simulink model "diagrama2_0"  (R2025a)
settings: Solver=ode4  StartTime=0.0  StopTime=20  FixedStep=1e-4  MaxStep=1e-3  RelTol=1e-3
InitFcn:
  | Np = 1;
  | Ns = 1;
  | Iscref = 1;
  | Voc = 1;
libraries: SignalEditorBlockLib x2, simulink x1
settings Model: Creator=BSLAY  LastModifiedBy=Rodri
settings SolverCC: InitialStep=1e-6
settings DebuggingCC: AlgebraicLoopMsg=none

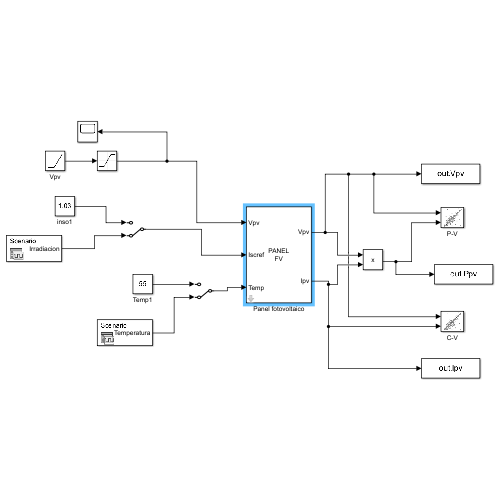
[thumbnail: Simulink's stored preview of the top-level diagram]
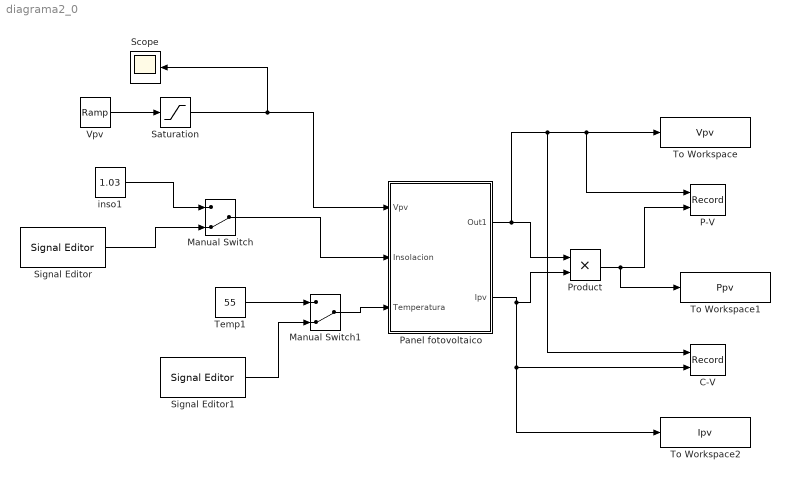
== system diagrama2_0 ==
  C-V : Record  NumPorts=2.0  FileSettingsInternal="{\"entries\":[{\"content\":{\"excelSettings\":{\"content\":{},\"type\":\"Streamout.ExcelSettings\"},\"parquetSettings\":{\"content\":{},\"type\":\"Streamout.ParquetSettings\"}},\"type\":\"Streamout.FileSettingStorage\",\"uuid\":\"\"}],\"packageUris\":[\"http:\\/\\/schema.mathworks.com\\/mf0\\/streamout_blocks\\/R2020a\"],\"version\":\"1.0\"}"  FrameSettings=[0, 0]  Layout=[1 1]  SignalsInternal="{\"entries\":[{\"content\":{\"signals\":[{\"content\":{\"blockPath\":[],\"dimensions\":[1],\"domain\":\"\",\"lineColor\":\"#7e2f8e\",\"lineWidth\":2,\"port\":1,\"sid\":[\"\"],\"signalID\":1,\"signalName\":\"Panel fotovoltaico:1\"},\"type\":\"RecordBlkView.Signal\",\"uuid\":\"\"},{\"content\":{\"blockPath\":[],\"dimensions\":[1],\"domain\":\"\",\"lineColor\":\"#77ac30\",\"lineWidth\":2,\"port\":2,\"sid\":[\"\"],\"signalID\":2,\"signalName\":\"Panel fotovoltaico:2\"},\"type\":\"RecordBlkView.Signal\",\"uuid\":\"\"}]},\"type\":\"RecordBlkView.InputSignals\",\"uuid\":\"\"}],\"packageUris\":[\"http:\\/\\/schema.mathworks.com\\/mf0\\/streamout_blocks\\/R2020a\"],\"version\":\"1.0\"}"  CompatibilityTag=XY
  Manual Switch : ManualSwitch  CurrentSetting=0
  Manual Switch1 : ManualSwitch  CurrentSetting=0
  P-V : Record  NumPorts=2.0  FileSettingsInternal="{\"entries\":[{\"content\":{\"excelSettings\":{\"content\":{},\"type\":\"Streamout.ExcelSettings\"},\"parquetSettings\":{\"content\":{},\"type\":\"Streamout.ParquetSettings\"}},\"type\":\"Streamout.FileSettingStorage\",\"uuid\":\"\"}],\"packageUris\":[\"http:\\/\\/schema.mathworks.com\\/mf0\\/streamout_blocks\\/R2020a\"],\"version\":\"1.0\"}"  FrameSettings=[0, 0]  Layout=[1 1]  SignalsInternal="{\"entries\":[{\"content\":{\"signals\":[{\"content\":{\"blockPath\":[],\"dimensions\":[1],\"domain\":\"\",\"lineColor\":\"#4dbeee\",\"lineWidth\":2,\"port\":1,\"sid\":[\"\"],\"signalID\":1,\"signalName\":\"Panel fotovoltaico:1\"},\"type\":\"RecordBlkView.Signal\",\"uuid\":\"\"},{\"content\":{\"blockPath\":[],\"dimensions\":[1],\"domain\":\"\",\"lineColor\":\"#a2142f\",\"lineWidth\":2,\"port\":2,\"sid\":[\"\"],\"signalID\":2,\"signalName\":\"Product\"},\"type\":\"RecordBlkView.Signal\",\"uuid\":\"\"}]},\"type\":\"RecordBlkView.InputSignals\",\"uuid\":\"\"}],\"packageUris\":[\"http:\\/\\/schema.mathworks.com\\/mf0\\/streamout_blocks\\/R2020a\"],\"version\":\"1.0\"}"  CompatibilityTag=XY
  Panel fotovoltaico : Subsystem  mask{Ns=36, Np=1, Corriente_en_corto_circuito=8.21, Voltaje_en_corto_circuito_abierto=37.3}
      mask prompts: Ns "Número de celdas en serie"; Np "Número de celdas en paralelo"; Corriente_en_corto_circuito "Iscref"; Voltaje_en_corto_circuito_abierto "Voc"
      mask Display:
      | disp('PANEL\nFV');
      | port_label('input', 1, 'Vpv');
      | port_label('input', 2, 'Iscref');
      | port_label('input', 3, 'Temp');
      | 
      | port_label('output', 1, 'Vpv');
      | port_label('output', 2, 'Ipv');
  Product : Product
  Saturation : Saturate  UpperLimit=40  LowerLimit=0
  Scope : Scope
      settings: ActiveDisplayYMinimum=-1  ActiveDisplayYMaximum=1
  Signal Editor : SignalEditorBlockLib/Signal Editor  FileName=Insolacion1.mat  ActiveScenario=Scenario  ActiveSignal=Irradiacion  IsBus=off  OutputBusObjectStr=Bus: BusObject  SampleTime=0  ZeroCross=off  OutputAfterFinalValue=Holding final value  Unit=W/m^2  PreserveSignalName=on  ApplySigPropsToAllScenarios=on  ApplySigPropsToAllSignals=off  SignalPropertySource=Dialog parameters
  Signal Editor1 : SignalEditorBlockLib/Signal Editor  FileName=Temperatura1.mat  ActiveScenario=Scenario  ActiveSignal=Temperatura  IsBus=off  OutputBusObjectStr=Bus: BusObject  SampleTime=0  ZeroCross=off  OutputAfterFinalValue=Holding final value  Unit=degC  PreserveSignalName=on  ApplySigPropsToAllScenarios=on  ApplySigPropsToAllSignals=off  SignalPropertySource=Dialog parameters
  Temp1 : Constant  Value=55
  To Workspace : ToWorkspace  VariableName=Vpv  SaveFormat=Timeseries  SampleTime=-1
  To Workspace1 : ToWorkspace  VariableName=Ppv  SaveFormat=Timeseries  SampleTime=-1
  To Workspace2 : ToWorkspace  VariableName=Ipv  SaveFormat=Timeseries  SampleTime=-1
  Vpv : simulink/Sources/Ramp  slope=-10/20  start=0  InitialOutput=10
  inso1 : Constant  Value=1.03
  wires:
  Manual Switch/1 -> Panel fotovoltaico/2(Insolacion)
  inso1/1 -> Manual Switch/1
  Manual Switch1/1 -> Panel fotovoltaico/3(Temperatura)
  Temp1/1 -> Manual Switch1/1
  Panel fotovoltaico/2(Ipv) -> To Workspace2/1, C-V/2, Product/2
  Panel fotovoltaico/1(Out1) -> C-V/1, P-V/1, To Workspace/1, Product/1
  Product/1 -> To Workspace1/1, P-V/2
  Signal Editor/1 -> Manual Switch/2
  Signal Editor1/1 -> Manual Switch1/2
  Vpv/1 -> Saturation/1
  Saturation/1 -> Scope/1, Panel fotovoltaico/1(Vpv)

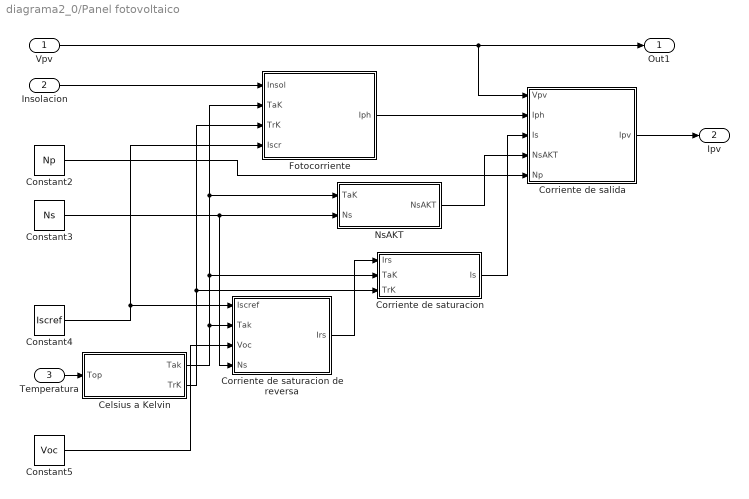
== system diagrama2_0/Panel fotovoltaico ==
  Vpv : Inport
  Insolacion : Inport  Port=2
  Temperatura : Inport  Port=3
  Celsius a Kelvin : Subsystem
  Constant2 : Constant  Value=Np
  Constant3 : Constant  Value=Ns
  Constant4 : Constant  Value=Iscref
  Constant5 : Constant  Value=Voc
  Corriente de salida : Subsystem
  Corriente de saturacion : Subsystem
  Corriente de saturacion de reversa : Subsystem
  Fotocorriente : Subsystem
  NsAKT : Subsystem
  Out1 : Outport
  Ipv : Outport  Port=2
  wires:
  Constant5/1 -> Corriente de saturacion de reversa/3(Voc)
  Corriente de salida/1(Ipv) -> Ipv/1
  Temperatura/1 -> Celsius a Kelvin/1(Top)
  Vpv/1 -> Corriente de salida/1(Vpv), Out1/1
  Fotocorriente/1(Iph) -> Corriente de salida/2(Iph)
  Insolacion/1 -> Fotocorriente/1(Insol)
  Constant3/1 -> Corriente de saturacion de reversa/4(Ns), NsAKT/2(Ns)
  Corriente de saturacion de reversa/1(Irs) -> Corriente de saturacion/1(Irs)
  Constant4/1 -> Corriente de saturacion de reversa/1(Iscref), Fotocorriente/4(Iscr)
  Constant2/1 -> Corriente de salida/5(Np)
  NsAKT/1(NsAKT) -> Corriente de salida/4(NsAKT)
  Corriente de saturacion/1(Is) -> Corriente de salida/3(Is)
  Celsius a Kelvin/1(Tak) -> Corriente de saturacion de reversa/2(Tak), Corriente de saturacion/2(TaK), NsAKT/1(TaK), Fotocorriente/2(TaK)
  Celsius a Kelvin/2(TrK) -> Corriente de saturacion/3(TrK), Fotocorriente/3(TrK)

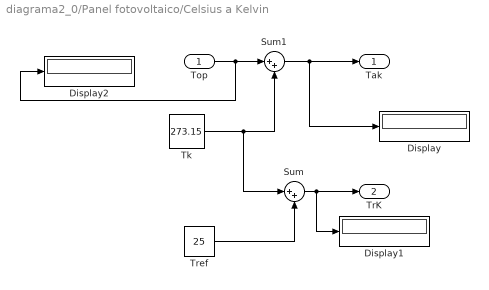
== system diagrama2_0/Panel fotovoltaico/Celsius a Kelvin ==
  Top : Inport
  Display : Display
  Display1 : Display
  Display2 : Display
  Sum : Sum  Inputs=|++
  Sum1 : Sum  Inputs=|++
  Tk : Constant  Value=273.15
  Tref : Constant  Value=25
  Tak : Outport
  TrK : Outport  Port=2
  wires:
  Sum/1 -> Display1/1, TrK/1
  Top/1 -> Display2/1, Sum1/1
  Tk/1 -> Sum/1, Sum1/2
  Sum1/1 -> Display/1, Tak/1
  Tref/1 -> Sum/2

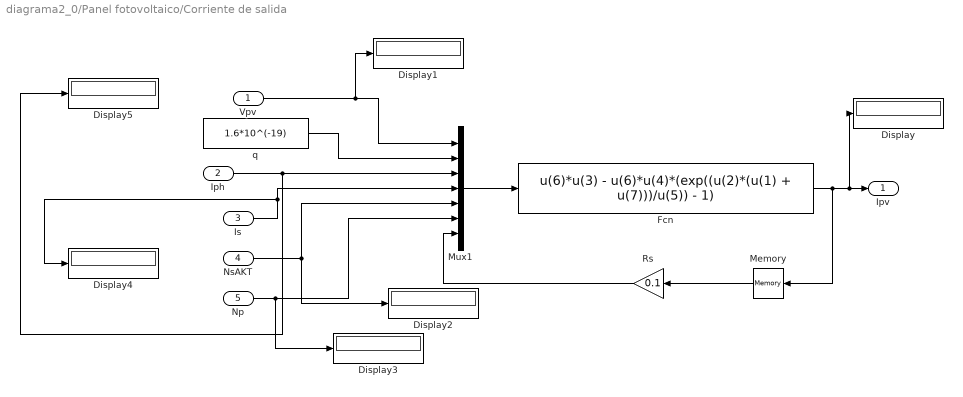
== system diagrama2_0/Panel fotovoltaico/Corriente de salida ==
  Vpv : Inport
  Iph : Inport  Port=2
  Is : Inport  Port=3
  NsAKT : Inport  Port=4
  Np : Inport  Port=5
  Display{,1..5} (6 alike) : Display
  "Fcn " : Fcn  Expr=u(6)*u(3) - u(6)*u(4)*(exp((u(2)*(u(1) + u(7)))/u(5)) - 1)
  Memory : Memory
  Mux1 : Mux  Inputs=7
  Rs : Gain  Gain=0.1
  q : Constant  Value=1.6*10^(-19)
  Ipv : Outport
  wires:
  "Fcn "/1 -> Memory/1, Display/1, Ipv/1
  q/1 -> Mux1/2
  Iph/1 -> Display5/1, Mux1/3
  Vpv/1 -> Display1/1, Mux1/1
  Mux1/1 -> "Fcn "/1
  Rs/1 -> Mux1/7
  NsAKT/1 -> Mux1/5, Display2/1
  Is/1 -> Display4/1, Mux1/4
  Np/1 -> Display3/1, Mux1/6
  Memory/1 -> Rs/1

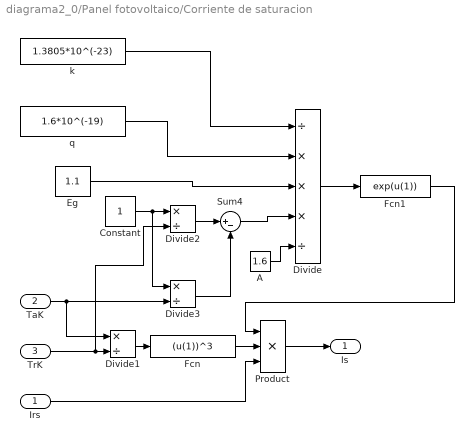
== system diagrama2_0/Panel fotovoltaico/Corriente de saturacion ==
  Irs : Inport
  TaK : Inport  Port=2
  TrK : Inport  Port=3
  A : Constant  Value=1.6
  "Constant " : Constant
  "Divide " : Product  Inputs=/***/
  "Divide1 " : Product  Inputs=*/
  "Divide2 " : Product  Inputs=*/
  "Divide3 " : Product  Inputs=*/
  Eg : Constant  Value=1.1
  "Fcn " : Fcn  Expr=(u(1))^3
  "Fcn1 " : Fcn  Expr=exp(u(1))
  "Product " : Product  Inputs=3
  Sum4 : Sum  Inputs=|+-
  k : Constant  Value=1.3805*10^(-23)
  q : Constant  Value=1.6*10^(-19)
  Is : Outport
  wires:
  "Divide1 "/1 -> "Fcn "/1
  "Divide2 "/1 -> Sum4/1
  q/1 -> "Divide "/2
  Eg/1 -> "Divide "/3
  TrK/1 -> "Divide2 "/2, "Divide1 "/2
  "Divide3 "/1 -> Sum4/2
  "Product "/1 -> Is/1
  A/1 -> "Divide "/5
  k/1 -> "Divide "/1
  "Divide "/1 -> "Fcn1 "/1
  TaK/1 -> "Divide1 "/1, "Divide3 "/2
  "Constant "/1 -> "Divide3 "/1, "Divide2 "/1
  Irs/1 -> "Product "/3
  "Fcn1 "/1 -> "Product "/1
  "Fcn "/1 -> "Product "/2
  Sum4/1 -> "Divide "/4

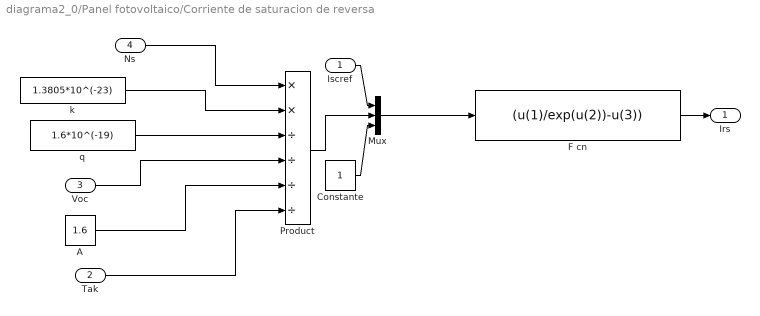
== system diagrama2_0/Panel fotovoltaico/Corriente de saturacion de reversa ==
  Iscref : Inport
  Tak : Inport  Port=2
  Voc : Inport  Port=3
  Ns : Inport  Port=4
  A : Constant  Value=1.6
  Constante : Constant
  F cn : Fcn  Expr=(u(1)/exp(u(2))-u(3))
  Mux : Mux  Inputs=3
  Product : Product  Inputs=**////
  k : Constant  Value=1.3805*10^(-23)
  q : Constant  Value=1.6*10^(-19)
  Irs : Outport
  wires:
  Iscref/1 -> Mux/1
  q/1 -> Product/3
  Ns/1 -> Product/1
  Tak/1 -> Product/6
  Voc/1 -> Product/4
  Product/1 -> Mux/2
  Constante/1 -> Mux/3
  A/1 -> Product/5
  k/1 -> Product/2
  F cn/1 -> Irs/1
  Mux/1 -> F cn/1

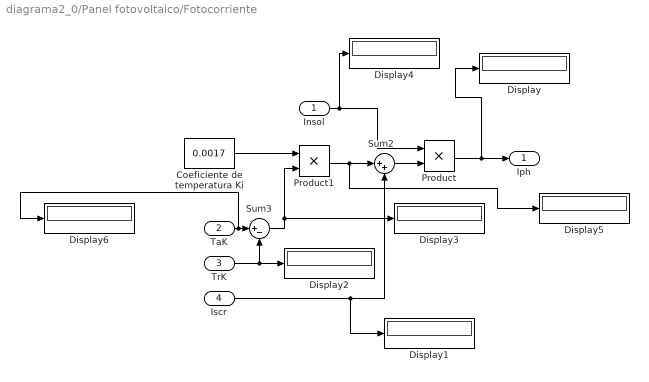
== system diagrama2_0/Panel fotovoltaico/Fotocorriente ==
  Insol : Inport
  TaK : Inport  Port=2
  TrK : Inport  Port=3
  Iscr : Inport  Port=4
  Coeficiente de temperatura Ki : Constant  Value=0.0017
  Display{,1..6} (7 alike) : Display
  Product : Product
  Product1 : Product
  Sum2 : Sum  Inputs=|++
  Sum3 : Sum  Inputs=|+-
  Iph : Outport
  wires:
  Insol/1 -> Display4/1, Product/1
  Coeficiente de temperatura Ki/1 -> Product1/1
  Product/1 -> Display/1, Iph/1
  Product1/1 -> Display5/1, Sum2/1
  TaK/1 -> Display6/1, Sum3/1
  Sum3/1 -> Product1/2, Display3/1
  TrK/1 -> Display2/1, Sum3/2
  Iscr/1 -> Display1/1, Sum2/2
  Sum2/1 -> Product/2

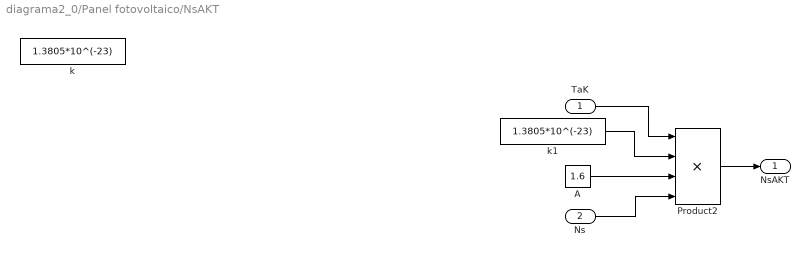
== system diagrama2_0/Panel fotovoltaico/NsAKT ==
  TaK : Inport
  Ns : Inport  Port=2
  A : Constant  Value=1.6
  Product2 : Product  Inputs=4
  k : Constant  Value=1.3805*10^(-23)
  k1 : Constant  Value=1.3805*10^(-23)
  NsAKT : Outport
  wires:
  Product2/1 -> NsAKT/1
  TaK/1 -> Product2/1
  k1/1 -> Product2/2
  A/1 -> Product2/3
  Ns/1 -> Product2/4
